simulink model "scheme"  (R2022b)
settings: Solver=FixedStepDiscrete  StartTime=0.0  StopTime=inf  RelTol=1e-3
libraries: dspmathops x9, dsparch4 x8, dspsnks4 x1, dspvision x1
settings Model: Creator=yungnik  LastModifiedBy=yungnik
settings SolverCC: AlgebraicLoopSolver=TrustRegion  AutoInsertRateTranBlk=on
settings DataIOCC: LimitDataPoints=on  SaveOutput=off  SignalLogging=off  SaveTime=off
settings OptimizationCC: LifeSpan=inf
settings DebuggingCC: AlgebraicLoopMsg=error  SingleTaskRateTransMsg=error  UnconnectedInputMsg=warning  UnconnectedOutputMsg=warning  UnconnectedLineMsg=warning  AllowSymbolicDim=off  SFUnexpectedBacktrackingDiag=warning  SFNoUnconditionalDefaultTransitionDiag=warning  SFExecutionAtInitializationDiag=none  SFMachineParentedDataDiag=warning  ArithmeticOperatorsInVariantConditions=warning
settings ModelReferenceCC: EnableRefExpFcnMdlSchedulingChecks=on
settings SFSimCC: SimUseLocalCustomCode=off  CustomCodeUndefinedFunction=UseInterfaceOnly
settings RTWCC: RTWUseLocalCustomCode=off
settings CodeAppCC: StateflowObjectComments=on
settings GRTTargetCC: TargetLangStandard=C89/C90 (ANSI)
settings ConfigComp: CovMetricSettings=dw  CovSaveCumulativeToWorkspaceVar=on  CovSaveSingleToWorkspaceVar=on  CovExternalEMLEnable=off  CovSFcnEnable=off

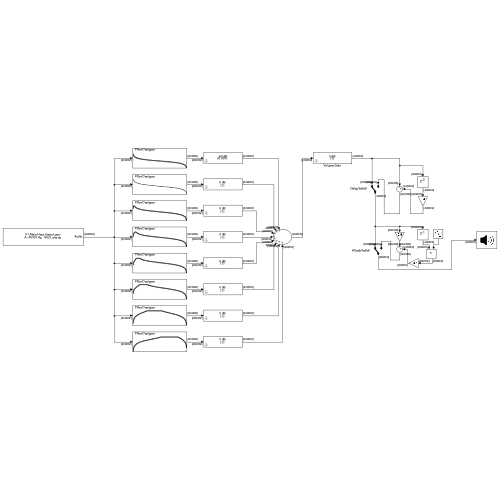
[thumbnail: Simulink's stored preview of the top-level diagram]
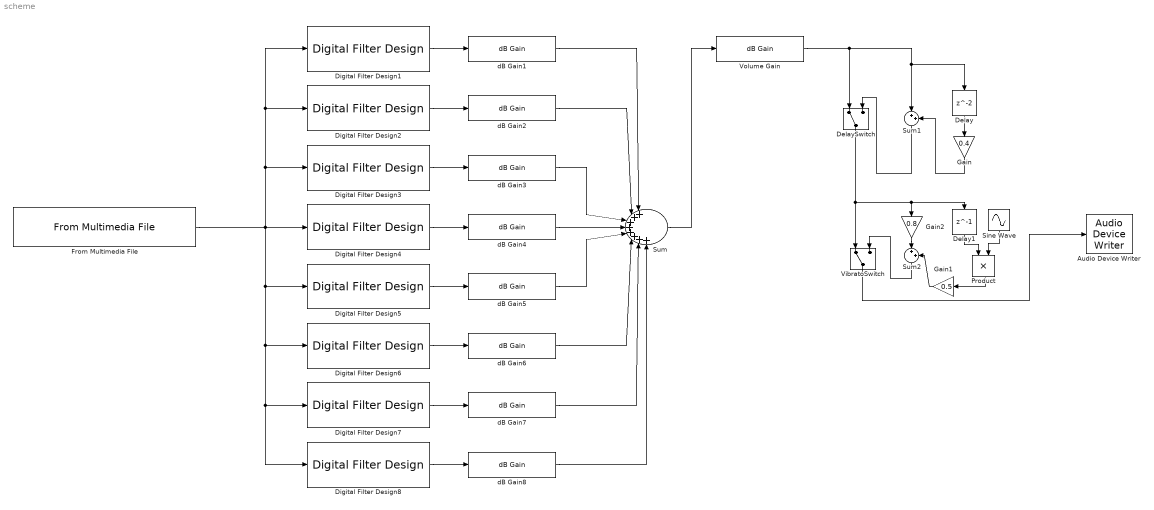
== system scheme ==
  Audio Device Writer : dspsnks4/Audio Device Writer  Driver=CoreAudio  Device=Динамики MacBook Air  InheritSampleRate=on  SampleRate=44100  BitDepth=16-bit integer  BufferSize=4096  NumBuffers=10  DefaultOutputChannelMapping=on  OutputChannelMapping=1:2  OutputNumUnderrunSamples=off  DriverIdx=5  DeviceWarnFlag=''
  Delay : Delay  InitialCondition=0
  Delay1 : Delay  DelayLength=1  InitialCondition=0
  DelaySwitch : ManualSwitch
  Digital Filter Design{1..8} (8 alike) : dsparch4/Digital Filter Design  mwdsp_browser_bugfix_var=off
  From Multimedia File : dspvision/From Multimedia File  inputFilename=/Users/yungnik/Downloads/01-Mein-Herz-brennt.wav  readRange=[1 Inf]  loop=on  numPlays=inf  outputStreams=Audio only  videoDataType=single  audioDataType=double  inheritSampleTime=on  userDefinedSampleTime=1/30  noAudioOutput=off  isIntensityVideo=off  fourcc=RGB  colorVideoFormat=Separate color signals  outputEOF=off  dataOrg=Column-major  audioFrameSize=4096  computeAudioFrameSize=off  outSamplingMode=Sample based
  Gain : Gain  Gain=0.4
  Gain1 : Gain  Gain=0.5
  Gain2 : Gain  Gain=0.8
  Product : Product
  Sine Wave : Sin  Frequency=50  SampleTime=0
  Sum : Sum  Inputs=|++++++++
  Sum1 : Sum  Inputs=|++
  Sum2 : Sum  Inputs=|++
  VibratoSwitch : ManualSwitch
  Volume Gain : dspmathops/dB Gain  dB=0  intype=Amplitude
  dB Gain1 : dspmathops/dB Gain  dB=-60  intype=Amplitude
  dB Gain{2..8} (7 alike) : dspmathops/dB Gain  dB=0  intype=Amplitude
  wires:
  From Multimedia File/1 -> Digital Filter Design8/1, Digital Filter Design7/1, Digital Filter Design6/1, Digital Filter Design5/1, Digital Filter Design1/1, Digital Filter Design2/1, Digital Filter Design3/1, Digital Filter Design4/1
  Digital Filter Design1/1 -> dB Gain1/1
  Digital Filter Design2/1 -> dB Gain2/1
  Digital Filter Design3/1 -> dB Gain3/1
  Digital Filter Design4/1 -> dB Gain4/1
  Digital Filter Design5/1 -> dB Gain5/1
  Digital Filter Design6/1 -> dB Gain6/1
  Digital Filter Design7/1 -> dB Gain7/1
  Digital Filter Design8/1 -> dB Gain8/1
  dB Gain1/1 -> Sum/1
  dB Gain2/1 -> Sum/2
  dB Gain3/1 -> Sum/3
  dB Gain4/1 -> Sum/4
  dB Gain5/1 -> Sum/5
  dB Gain6/1 -> Sum/6
  dB Gain7/1 -> Sum/7
  dB Gain8/1 -> Sum/8
  Sum/1 -> Volume Gain/1
  Volume Gain/1 -> DelaySwitch/1, Sum1/1, Delay/1
  Delay/1 -> Gain/1
  Gain/1 -> Sum1/2
  Sum1/1 -> DelaySwitch/2
  DelaySwitch/1 -> VibratoSwitch/1, Delay1/1, Gain2/1
  Sum2/1 -> VibratoSwitch/2
  VibratoSwitch/1 -> Audio Device Writer/1
  Gain2/1 -> Sum2/1
  Delay1/1 -> Product/1
  Sine Wave/1 -> Product/2
  Product/1 -> Gain1/1
  Gain1/1 -> Sum2/2
